simulink model "motion_sim_lonlat"  (R2020a)
settings: Solver=ode4  StartTime=0.0  StopTime=20  FixedStep=Tc  RelTol=1e-3
values from neighbouring files (symbols this model uses):
  delta_ref = 10*pi/180    (= 0.174532925199)    [para_set.m]
  Ki = 0.01    [para_set.m]
  Kp = 1    [para_set.m]
  tau = 0.8    [para_set.m]
  V_ref = 30    [para_set.m]
  vx_ini = 30    [para_set.m]
  vy_ini = 0    [para_set.m]
  X_ini = 0    [para_set.m]
  Y_ini = 0    [para_set.m]
  yaw_ini = 0    [para_set.m]
  yawrate_ini = 0    [para_set.m]
undefined symbols (not defined in the file or in its folder): global_motion, vehicle_motion, vehicle_motion_nonlinear
settings Model: Creator=Mook  LastModifiedBy=Mook
settings DataIOCC: ReturnWorkspaceOutputs=off

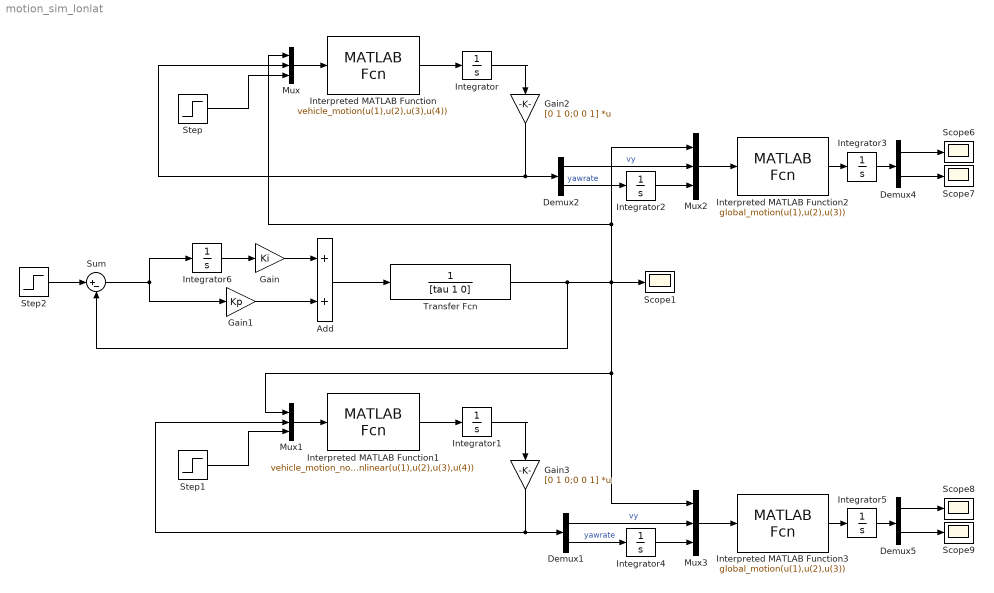
== system motion_sim_lonlat ==
  Add : Sum
  Demux{1..2,4..5} (4 alike) : Demux  Outputs=2
  Gain : Gain  Gain=Ki
  Gain1 : Gain  Gain=Kp
  Gain2 : Gain  Gain=[0 1 0;0 0 1]  Multiplication=Matrix(K*u)
  Gain3 : Gain  Gain=[0 1 0;0 0 1]  Multiplication=Matrix(K*u)
  Integrator : Integrator  InitialCondition=[vx_ini; vy_ini; yawrate_ini]
  Integrator1 : Integrator  InitialCondition=[vx_ini vy_ini yawrate_ini]
  Integrator2 : Integrator  InitialCondition=[yaw_ini]
  Integrator3 : Integrator  InitialCondition=[X_ini Y_ini]
  Integrator4 : Integrator  InitialCondition=[yaw_ini]
  Integrator5 : Integrator  InitialCondition=[X_ini Y_ini]
  Integrator6 : Integrator
  Interpreted MATLAB Function : MATLABFcn  MATLABFcn=vehicle_motion(u(1),u(2),u(3),u(4))  OutputDimensions=3
  Interpreted MATLAB Function1 : MATLABFcn  MATLABFcn=vehicle_motion_nonlinear(u(1),u(2),u(3),u(4))  OutputDimensions=3
  Interpreted MATLAB Function2 : MATLABFcn  MATLABFcn=global_motion(u(1),u(2),u(3))  OutputDimensions=2
  Interpreted MATLAB Function3 : MATLABFcn  MATLABFcn=global_motion(u(1),u(2),u(3))  OutputDimensions=2
  Mux{,1..3} (4 alike) : Mux  Inputs=3
  Scope{1,6..9} (5 alike) : Scope
  Step : Step  Time=2  After=delta_ref  SampleTime=0
  Step1 : Step  Time=2  After=delta_ref  SampleTime=0
  Step2 : Step  Time=10  Before=5  After=V_ref  SampleTime=0
  Sum : Sum  Inputs=|+-
  Transfer Fcn : TransferFcn  Denominator=[tau 1 0]
  wires:
  Mux/1 -> Interpreted MATLAB Function/1
  Interpreted MATLAB Function/1 -> Integrator/1
  Integrator/1 -> Gain2/1
  Interpreted MATLAB Function1/1 -> Integrator1/1
  Integrator1/1 -> Gain3/1
  Mux1/1 -> Interpreted MATLAB Function1/1
  Integrator2/1 -> Mux2/3
  Mux2/1 -> Interpreted MATLAB Function2/1
  Interpreted MATLAB Function2/1 -> Integrator3/1
  Integrator3/1 -> Demux4/1
  Demux1/2 -> Integrator4/1  "yawrate"
  Mux3/1 -> Interpreted MATLAB Function3/1
  Integrator5/1 -> Demux5/1
  Integrator4/1 -> Mux3/3
  Interpreted MATLAB Function3/1 -> Integrator5/1
  Demux1/1 -> Mux3/2  "vy"
  Demux4/1 -> Scope6/1
  Demux4/2 -> Scope7/1
  Demux5/1 -> Scope8/1
  Demux5/2 -> Scope9/1
  Integrator6/1 -> Gain/1
  Gain1/1 -> Add/2
  Gain/1 -> Add/1
  Add/1 -> Transfer Fcn/1
  Sum/1 -> Gain1/1, Integrator6/1
  Step2/1 -> Sum/1
  Transfer Fcn/1 -> Sum/2, Mux1/1, Mux3/1, Mux/1, Mux2/1, Scope1/1
  Step1/1 -> Mux1/3
  Step/1 -> Mux/3
  Demux2/1 -> Mux2/2  "vy"
  Demux2/2 -> Integrator2/1  "yawrate"
  Gain2/1 -> Demux2/1, Mux/2
  Gain3/1 -> Demux1/1, Mux1/2
